simulink model "clark_park_trans"  (R2022a)
settings: Solver=VariableStepDiscrete  StartTime=0.0  StopTime=10.0  MaxStep=5e-05  RelTol=1e-3
libraries: simulink x1, spspowerguiLib x1
settings Model: Creator=XieXW  LastModifiedBy=XieXW

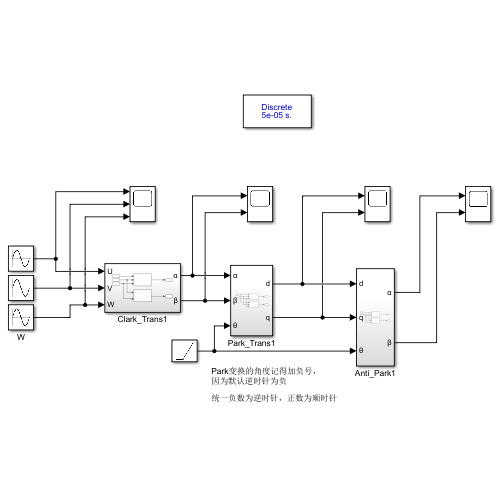
[thumbnail: Simulink's stored preview of the top-level diagram]
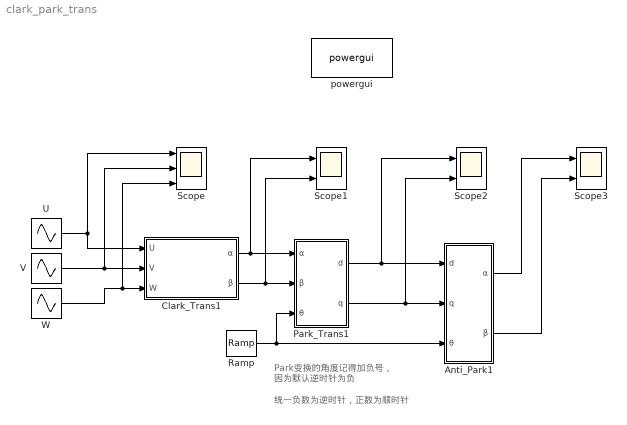
== system clark_park_trans ==
  note: 统一负数为逆时针，正数为顺时针
  note: Park变换的角度记得加负号，
      | 因为默认逆时针为负
  Anti_Park1 : Subsystem
  Clark_Trans1 : Subsystem
  Park_Trans1 : Subsystem
  Ramp : simulink/Sources/Ramp  slope=pi/2  start=0  InitialOutput=0
  Scope : Scope  NumInputPorts=3
  Scope1 : Scope  NumInputPorts=2
  Scope2 : Scope  NumInputPorts=2
  Scope3 : Scope  NumInputPorts=2
  U : Sin  Frequency=pi/2  SampleTime=0
  V : Sin  Frequency=pi/2  Phase=-2*pi/3  SampleTime=0
  W : Sin  Frequency=pi/2  Phase=2*pi/3  SampleTime=0
  powergui : spspowerguiLib/powergui  Priority=1  SimulationMode=Discrete  SampleTime=50e-6  frequency=60  Iterations=50  frequencyindice=0  Pbase=100e6  ErrMax=1e-4  UnitsV=kV  UnitsW=MW  buscounter=0  FunctionMessages=off  echomessages=off  EnableUseOfTLC=off  CurrentSourceSwitches=off  DisableSnubberDevices=off  DisableRonSwitches=off  DisableVfSwitches=off  DisplayEquations=off  AutomaticDiscreteSolvers=off  SolverType=Tustin/Backward Euler (TBE)  Interpol=off  ExternalGateDelay=off  methode=off  Ts=100  x0status=blocks  SPID=on  SwTol=0  HookPort=off  NonlinearTolerance=1e-4  nMaxIteration=100  ContinueOnMaxIteration=off  RestoreLinks=warning  ResistiveCurrentMeasurement=off  Frange=[0:2:500]  Ylog=off  Xlog=on  ShowGrid=off  save=off  variable=ZData  structure=0  ZoomFFT=off  StartTime=0.0  cycles=1  DisplayStyle=1  fundamental=60  FreqAxis=off  MaxFrequency=1000  frequencyindicesteady=1  RmsSteady=1  display=off
  wires:
  U/1 -> Scope/1, Clark_Trans1/1(U)
  V/1 -> Clark_Trans1/2(V), Scope/2
  W/1 -> Scope/3, Clark_Trans1/3(W)
  Clark_Trans1/1(α) -> Scope1/1, Park_Trans1/1(α)
  Clark_Trans1/2(β) -> Scope1/2, Park_Trans1/2(β)
  Ramp/1 -> Park_Trans1/3(θ), Anti_Park1/3(θ)
  Park_Trans1/1(d) -> Scope2/1, Anti_Park1/1(d)
  Park_Trans1/2(q) -> Scope2/2, Anti_Park1/2(q)
  Anti_Park1/1(α) -> Scope3/1
  Anti_Park1/2(β) -> Scope3/2

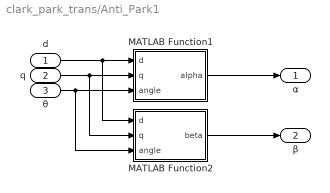
== system clark_park_trans/Anti_Park1 ==
  d : Inport
  q : Inport  Port=2
  θ : Inport  Port=3
  MATLAB Function1 : MATLAB Function  TreatAsAtomicUnit=on
  MATLAB Function2 : MATLAB Function  TreatAsAtomicUnit=on
  α : Outport
  β : Outport  Port=2
  wires:
  MATLAB Function1/1(alpha) -> α/1
  d/1 -> MATLAB Function2/1(d), MATLAB Function1/1(d)
  q/1 -> MATLAB Function2/2(q), MATLAB Function1/2(q)
  θ/1 -> MATLAB Function2/3(angle), MATLAB Function1/3(angle)
  MATLAB Function2/1(beta) -> β/1

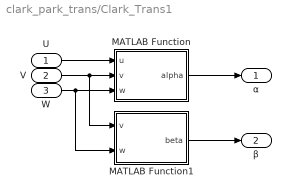
== system clark_park_trans/Clark_Trans1 ==
  U : Inport
  V : Inport  Port=2
  W : Inport  Port=3
  MATLAB Function : MATLAB Function  TreatAsAtomicUnit=on
  MATLAB Function1 : MATLAB Function  TreatAsAtomicUnit=on
  α : Outport
  β : Outport  Port=2
  wires:
  U/1 -> MATLAB Function/1(u)
  V/1 -> MATLAB Function1/1(v), MATLAB Function/2(v)
  W/1 -> MATLAB Function1/2(w), MATLAB Function/3(w)
  MATLAB Function/1(alpha) -> α/1
  MATLAB Function1/1(beta) -> β/1

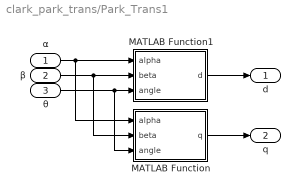
== system clark_park_trans/Park_Trans1 ==
  α : Inport
  β : Inport  Port=2
  θ : Inport  Port=3
  MATLAB Function : MATLAB Function  TreatAsAtomicUnit=on
  MATLAB Function1 : MATLAB Function  TreatAsAtomicUnit=on
  d : Outport
  q : Outport  Port=2
  wires:
  α/1 -> MATLAB Function/1(alpha), MATLAB Function1/1(alpha)
  MATLAB Function1/1(d) -> d/1
  β/1 -> MATLAB Function/2(beta), MATLAB Function1/2(beta)
  MATLAB Function/1(q) -> q/1
  θ/1 -> MATLAB Function/3(angle), MATLAB Function1/3(angle)

== matlab function clark_park_trans/Anti_Park1/MATLAB Function2 ==
  data: d input; beta output; q input; angle input
function beta = fcn(d,q,angle)

beta = d*sin(angle)+q*cos(angle);

== matlab function clark_park_trans/Clark_Trans1/MATLAB Function ==
  data: u input; alpha output; v input; w input
function alpha = fcn(u,v,w)

alpha = (2/3)*(u+(-1/2)*v+(-1/2)*w);

== matlab function clark_park_trans/Clark_Trans1/MATLAB Function1 ==
  data: beta output; v input; w input
function beta = fcn(v,w)

beta = (2/3)*((sqrt(3)/2)*v+(-sqrt(3)/2)*w);

== matlab function clark_park_trans/Park_Trans1/MATLAB Function ==
  data: alpha input; q output; beta input; angle input
function q = fcn(alpha,beta,angle)

q = -alpha*sin(angle)+beta*cos(angle);

== matlab function clark_park_trans/Park_Trans1/MATLAB Function1 ==
  data: alpha input; d output; beta input; angle input
function d = fcn(alpha,beta,angle)

d = alpha*cos(angle)+beta*sin(angle);

== matlab function clark_park_trans/Anti_Park1/MATLAB Function1 ==
  data: d input; alpha output; q input; angle input
function alpha = fcn(d,q,angle)

alpha = d*cos(angle)-q*sin(angle);
